simulink model "Lab4_astatyczny"  (R2020b)
settings: Solver=VariableStepAuto  StartTime=0.0  StopTime=10.0  RelTol=1e-3
values from neighbouring files (symbols this model uses):
  SP = 0.5    [LAB4.m]
  T = 45    [LAB4.m]
  tau = 22    [LAB4.m]
undefined symbols (not defined in the file or in its folder): h
settings Model: Creator=Maciek  LastModifiedBy=Maciek

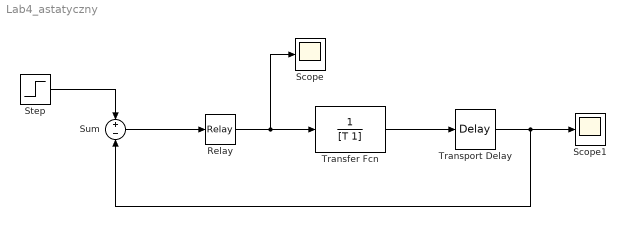
== system Lab4_astatyczny ==
  Relay : Relay  OnSwitchValue=h  OffSwitchValue=-h
  Scope : Scope
  Scope1 : Scope
  Step : Step  After=SP  SampleTime=0
  Sum : Sum  Inputs=+-
  Transfer Fcn : TransferFcn  Denominator=[T 1]
  Transport Delay : TransportDelay  DelayTime=tau  PadeOrder=10
  wires:
  Relay/1 -> Scope/1, Transfer Fcn/1
  Transfer Fcn/1 -> Transport Delay/1
  Transport Delay/1 -> Sum/2, Scope1/1
  Step/1 -> Sum/1
  Sum/1 -> Relay/1
